simulink model "DragBlock_V5"  (R2022b)
settings: Solver=VariableStepAuto  StartTime=0.0  StopTime=10.0  RelTol=1e-3
settings Model: Creator=antonisioannou  LastModifiedBy=antonisioannou
settings ModelReferenceCC: EnableRefExpFcnMdlSchedulingChecks=on

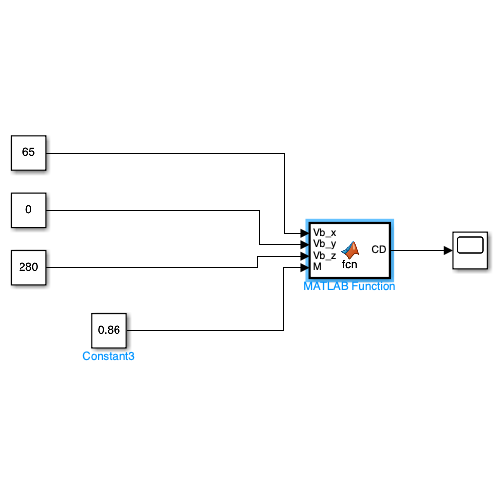
[thumbnail: Simulink's stored preview of the top-level diagram]
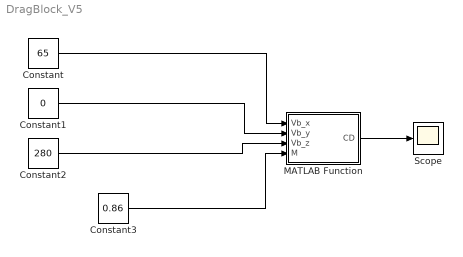
== system DragBlock_V5 ==
  Constant : Constant  Value=65
  Constant1 : Constant  Value=0
  Constant2 : Constant  Value=280
  Constant3 : Constant  Value=0.86
  MATLAB Function : MATLAB Function  TreatAsAtomicUnit=on
  Scope : Scope
  wires:
  Constant3/1 -> MATLAB Function/4(M)
  Constant2/1 -> MATLAB Function/3(Vb_z)
  Constant1/1 -> MATLAB Function/2(Vb_y)
  Constant/1 -> MATLAB Function/1(Vb_x)
  MATLAB Function/1(CD) -> Scope/1

== matlab function DragBlock_V5/MATLAB Function ==
  data: Vb_x input; Vb_y input; Vb_z input; M input; CD output
function CD = fcn( Vb_x, Vb_y, Vb_z,M)
%% Function takes as inputs Mach number and all velocities on vector form 

% Dimensions
M=0.86
L=4.48;  % body legth 
b=0.566; %Distance from fin-tip to fin-tip  %fin height (24)
d= 0.194; %Body diameters
f= L/d ; %Finess ratio
N_f= 3; % Number of fins
C_R=0.3 ;   %Root fin chord
S_f=N_f*(0.42+0.2)*0.24/2 %Fin Surface Area 
Nose_coneArea=0.23;
Rs= 5*10^-6  ;  % surface roughness
A_T=2.1834+0.23;   % total area
Aref=2.1834+0.23   ;  %reference area

Awet_fins=0.078*3  % fin wetted area 
Awet_body=2.1834+0.23;

d1= 0.194 ;     % diameter at the beginning of boattail 
d2=0.11 ;      % diameter at the end of the boattail (end of the rocket)
Abase=0.0043 ;   %Area at the end of the rocket 
Aboat=0.0804 ;     %Area at the start of the boattail
gamma=1/(d1-d2); % factor definning boattail profile 
Fin_thetaLE=53;   % Fin leading edge angle 
Re=81.6e06;
Rcrit=52*(Rs/L)^(-1.039);
t_f=0.003;
t_c=0.0123;

c_tip_can=0.045;
c_chord_can=0.07;
c_tip_fins=0.15;
c_chord_fins=0.322;
Awet_can= 0.007*3 % canards wetted area

%% Mean aerodynamic chord for fins 
lamda_fins=(c_tip_fins/c_chord_fins);
cbar_fins=2/3*c_chord_fins*(1+lamda_fins+(lamda_fins)^2)/(1+lamda_fins);






%%  Mean aerodynamic chord calc for canards.
lamda_can=(c_tip_can/c_chord_can);      % taper ratio canards 

cbar_can=2/3*c_chord_can*(1+lamda_can+(lamda_can)^2)/(1+lamda_can);



%%

if Re < 10E04
    Cf=1.48*10^-2;

elseif (10^3<Re) && (Re<Rcrit) 
Cf=1/(1.5*log(Re)-5.6)^2;

else 
    Cf=0.032*(Rs/L)^0.2;

end

% Cf comdepress. corrwedwedection
Cf=Cf*(1-0.1*M^2)

% CD  due to skin friction of rocket calc.
CD_friction=Cf*((1+1/(2*f))*Awet_body+(1+2*t_f/cbar_fins)*Awet_fins + (1+2*t_c/cbar_can)*Awet_can)/Aref

%  pressure drag 
CDbase=0.12+0.13*M^2 % due to base drag

% The following are for calculating the pressure drag, due to the boattail
if gamma<1
    factor=1;
elseif (1<gamma) && (gamma<3)
factor=(3-gamma)/3;
elseif gamma>3
    factor=0;
end
%boattail press. drag 
CD_boat=Abase/Aboat*CDbase*factor; 

%Stagnation Pressure DRAG
CDP_0=((1-M^2)^(-0.417)-1)

% Fin pressure drag 
CDfin=CDP_0*(cos(Fin_thetaLE))^2; % For M<0.9

% Drag cerff. launch guide
%CD_parasitic=max([1.3-0.3*L/d,1])*CDP_0;

%Total zero lift drag 

%CD=(CDbase+CD_boat+CDfin+CD_parasitic)*A_T/Aref + CD_friction
CD=(CDbase+CD_boat+CDfin)*A_T/Aref + CD_friction
end
